simulink model "controller_dev_sg"  (R2018b)
settings: configuration reference "Physics" (kept outside this file)
model workspace (MAT data in the model file):
  m = 1000
undefined symbols (not defined in the file or in its folder): C, P_MLOC_NumberOfNoSendFrames, tS, TUMHealthStatus, TUMStateEstimationState, TUMVehicleState, x0_vehiclepose_stm
libraries: xpcrtudplib x13, simulink x12, canmsglib x12, etargetslib x10, speedgoatlib_IO614 x9, misc x4, xpcutilitieslib x1
(part 1 of 2)
settings Model: DataDictionary=controller_dev_sg.sldd  sg_rtwmakecfg_data=_sglibc__IO61X_Library_  PauseTimes=9.280  Creator=wischnewski  LastModifiedBy=ge34qer

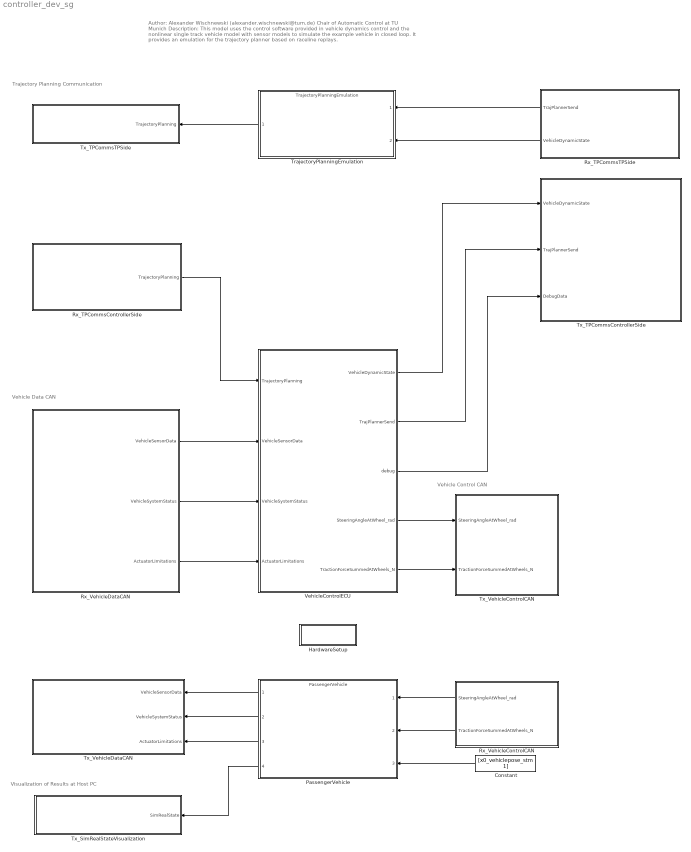
== system controller_dev_sg ==
  note: Visualization of Results at Host PC
  note: Trajectory Planning Communication
  note: Vehicle Control CAN
  note: Vehicle Data CAN
  note: Author: Alexander Wischnewski (alexander.wischnewski@tum.de)
      | Chair of Automatic Control at TU Munich
      |
      | Description: This model uses the control software provided in vehicle dynamics control and the nonlinear single track vehicle model
      | with sensor models to simulate the example vehicle in closed loop. It provides an emulation for the trajectory planner based on raceline replays.
  Constant : Constant  Value=[x0_vehiclepose_stm 1]
  HardwareSetup : Subsystem
  PassengerVehicle : ModelReference  ModelNameDialog=PassengerVehicle  SimulationMode=Normal  ModelReferenceVersion=1.770
  Rx_TPCommsControllerSide : Subsystem
  Rx_TPCommsTPSide : Subsystem
  Rx_VehicleControlCAN : Subsystem
  Rx_VehicleDataCAN : Subsystem
  TrajectoryPlanningEmulation : ModelReference  ModelNameDialog=TrajectoryPlanningEmulation.slx  SimulationMode=Normal  ModelReferenceVersion=1.722
  Tx_SimRealStateVisualization : Subsystem
  Tx_TPCommsControllerSide : Subsystem
  Tx_TPCommsTPSide : Subsystem
  Tx_VehicleControlCAN : Subsystem
  Tx_VehicleDataCAN : Subsystem
  VehicleControlECU : Subsystem
  wires:
  VehicleControlECU/3(debug) -> Tx_TPCommsControllerSide/3(DebugData)
  Rx_TPCommsControllerSide/1(TrajectoryPlanning) -> VehicleControlECU/1(TrajectoryPlanning)
  VehicleControlECU/1(VehicleDynamicState) -> Tx_TPCommsControllerSide/1(VehicleDynamicState)
  VehicleControlECU/2(TrajPlannerSend) -> Tx_TPCommsControllerSide/2(TrajPlannerSend)
  Rx_TPCommsTPSide/1(TrajPlannerSend) -> TrajectoryPlanningEmulation/1
  Rx_TPCommsTPSide/2(VehicleDynamicState) -> TrajectoryPlanningEmulation/2
  TrajectoryPlanningEmulation/1 -> Tx_TPCommsTPSide/1(TrajectoryPlanning)
  VehicleControlECU/4(SteeringAngleAtWheel_rad) -> Tx_VehicleControlCAN/1(SteeringAngleAtWheel_rad)
  VehicleControlECU/5(TractionForceSummedAtWheels_N) -> Tx_VehicleControlCAN/2(TractionForceSummedAtWheels_N)
  Rx_VehicleControlCAN/1(SteeringAngleAtWheel_rad) -> PassengerVehicle/1
  Rx_VehicleControlCAN/2(TractionForceSummedAtWheels_N) -> PassengerVehicle/2
  PassengerVehicle/1 -> Tx_VehicleDataCAN/1(VehicleSensorData)
  PassengerVehicle/2 -> Tx_VehicleDataCAN/2(VehicleSystemStatus)
  PassengerVehicle/3 -> Tx_VehicleDataCAN/3(ActuatorLimitations)
  Rx_VehicleDataCAN/3(ActuatorLImitations) -> VehicleControlECU/4(ActuatorLimitations)
  Rx_VehicleDataCAN/2(VehicleSystemStatus) -> VehicleControlECU/3(VehicleSystemStatus)
  Rx_VehicleDataCAN/1(VehicleSensorData) -> VehicleControlECU/2(VehicleSensorData)
  PassengerVehicle/4 -> Tx_SimRealStateVisualization/1(SimRealState)
  Constant/1 -> PassengerVehicle/3

== system controller_dev_sg/HardwareSetup ==
  CAN & LIN Setup : speedgoatlib_IO614/CAN & LIN Setup  id=1  drLtr=C:  PCISlot=-1  port1=CAN (HS/LS)  port2=CAN (HS)  port3=CAN (HS)  port4=CAN (HS)  opModeCAN1=Highspeed (HS)  bdrCAN1=1 MBaud  usrBdrCAN1=[5, 1, 13, 2]  stdAccMaskCAN1=[0, 0]  extAccMaskCAN1=[0, 0]  opModeCAN2=Highspeed (HS)  bdrCAN2=1 MBaud  usrBdrCAN2=[5, 1, 13, 2]  stdAccMaskCAN2=[0, 0]  extAccMaskCAN2=[0, 0]  opModeCAN3=Highspeed (HS)  bdrCAN3=1 MBaud  usrBdrCAN3=[5, 1, 13, 2]  stdAccMaskCAN3=[0, 0]  extAccMaskCAN3=[0, 0]  opModeCAN4=Highspeed (HS)  bdrCAN4=1 MBaud  usrBdrCAN4=[5, 1, 13, 2]  stdAccMaskCAN4=[0, 0]  extAccMaskCAN4=[0, 0]  initStruct=[]  termStruct=[]  opModeLIN=Master  bdrLIN=19200  protl=IO614  qtyMod=1  chNo=[1, 2, 3, 4]  ptTypes=[1, 1, 1, 1, 2]  protlHelpIdx=[0, 1, 2, 3, 0]  isFDMod=0  drvLtr=C:  opModeLIN2=Master  bdrLIN2=19200
      settings: SourceProductName=Simulink Real-Time: Speedgoat Library
  "Real-time UDP Configuration " : xpcrtudplib/UDP Configure  Priority=1  IpAddress=10.0.1.0  SubnetMask=255.255.255.0  Gateway=0.0.0.0  PciBus=14  PciSlot=0  PciFunction=0  ID=3  tune=0  disable=off  enableMulticast=off  MulticastIpAddress={}  MulticastMask={}
      settings: SourceProductName=Simulink Real-Time  SourceProductBaseCode=XP
  Real-time UDP Configuration 1 : xpcrtudplib/UDP Configure  Priority=1  IpAddress=10.0.2.0  SubnetMask=255.255.255.0  Gateway=0.0.0.0  PciBus=16  PciSlot=0  PciFunction=0  ID=3  tune=0  disable=off  enableMulticast=off  MulticastIpAddress={}  MulticastMask={}
      settings: SourceProductName=Simulink Real-Time  SourceProductBaseCode=XP

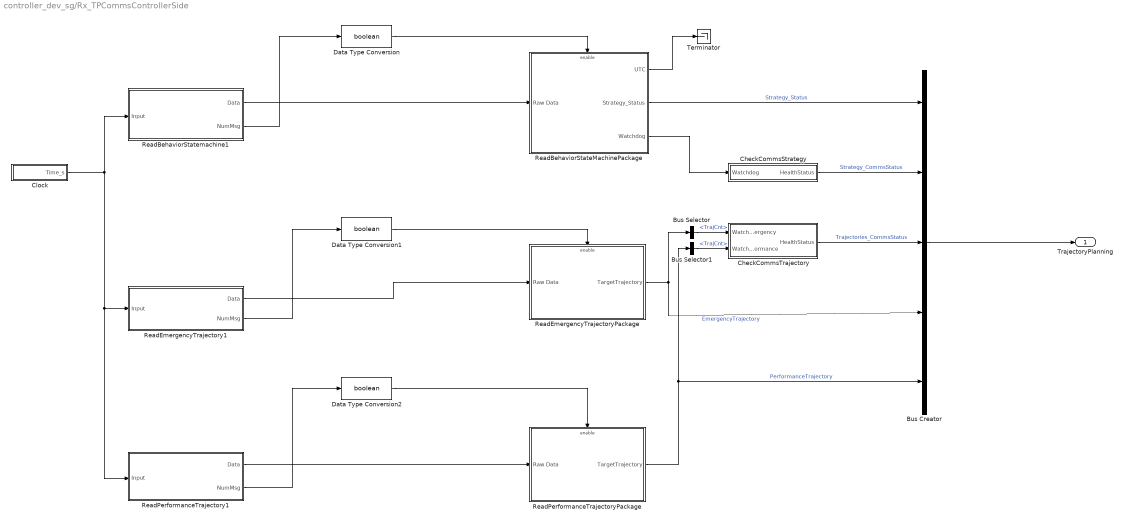
== system controller_dev_sg/Rx_TPCommsControllerSide ==
  Bus Creator : BusCreator  Inputs=5
  Bus Selector : BusSelector  OutputSignals=TrajCnt
  Bus Selector1 : BusSelector  OutputSignals=TrajCnt
  CheckCommsStrategy : Subsystem
  CheckCommsTrajectory : Subsystem
  Clock : Subsystem
  Data Type Conversion : DataTypeConversion  OutDataTypeStr=boolean
  Data Type Conversion1 : DataTypeConversion  OutDataTypeStr=boolean
  Data Type Conversion2 : DataTypeConversion  OutDataTypeStr=boolean
  ReadBehaviorStateMachinePackage : Subsystem  Priority=1000
  ReadBehaviorStatemachine1 : Subsystem  Priority=1
  ReadEmergencyTrajectory1 : Subsystem  Priority=1000
  ReadEmergencyTrajectoryPackage : Subsystem  Priority=1000
  ReadPerformanceTrajectory1 : Subsystem  Priority=1000
  ReadPerformanceTrajectoryPackage : Subsystem  Priority=1000
  Terminator : Terminator
  TrajectoryPlanning : Outport  OutDataTypeStr=Bus: TrajectoryPlanning  BusOutputAsStruct=on
  wires:
  ReadBehaviorStateMachinePackage/1(UTC) -> Terminator/1
  ReadPerformanceTrajectoryPackage/1(TargetTrajectory) -> Bus Selector1/1, Bus Creator/5  "PerformanceTrajectory"
  Clock/1(Time_s) -> ReadPerformanceTrajectory1/1(Input), ReadEmergencyTrajectory1/1(Input), ReadBehaviorStatemachine1/1(Input)
  CheckCommsTrajectory/1(HealthStatus) -> Bus Creator/3  "Trajectories_CommsStatus"
  ReadBehaviorStateMachinePackage/2(Strategy_Status) -> Bus Creator/1  "Strategy_Status"
  CheckCommsStrategy/1(HealthStatus) -> Bus Creator/2  "Strategy_CommsStatus"
  ReadEmergencyTrajectoryPackage/1(TargetTrajectory) -> Bus Creator/4, Bus Selector/1  "EmergencyTrajectory"
  Bus Selector/1 -> CheckCommsTrajectory/1(WatchdogEmergency)  "<TrajCnt>"
  Bus Selector1/1 -> CheckCommsTrajectory/2(WatchdogPerformance)  "<TrajCnt>"
  ReadBehaviorStateMachinePackage/3(Watchdog) -> CheckCommsStrategy/1(Watchdog)
  ReadEmergencyTrajectory1/2(NumMsg) -> Data Type Conversion1/1
  ReadEmergencyTrajectory1/1(Data) -> ReadEmergencyTrajectoryPackage/1(Raw Data)
  ReadPerformanceTrajectory1/1(Data) -> ReadPerformanceTrajectoryPackage/1(Raw Data)
  ReadPerformanceTrajectory1/2(NumMsg) -> Data Type Conversion2/1
  ReadBehaviorStatemachine1/2(NumMsg) -> Data Type Conversion/1
  ReadBehaviorStatemachine1/1(Data) -> ReadBehaviorStateMachinePackage/1(Raw Data)
  Data Type Conversion/1 -> ReadBehaviorStateMachinePackage/Enable
  Data Type Conversion1/1 -> ReadEmergencyTrajectoryPackage/Enable
  Data Type Conversion2/1 -> ReadPerformanceTrajectoryPackage/Enable
  Bus Creator/1 -> TrajectoryPlanning/1

== system controller_dev_sg/Rx_TPCommsTPSide ==
  Bus Creator : BusCreator  Inputs=2
  Data Type Conversion : DataTypeConversion  OutDataTypeStr=boolean
  Data Type Conversion1 : DataTypeConversion  OutDataTypeStr=boolean
  ReadBehaviorStateMachine : Subsystem  Priority=1000
  ReadBehaviorStateMachinePackage : Subsystem  Priority=1000
  ReadTrajectoryGeneration : Subsystem  Priority=1000
  ReadTrajectoryGeneration1 : Subsystem  Priority=1000
  Subsystem : Subsystem
  Terminator : Terminator
  TrajPlannerSend : Outport  OutDataTypeStr=Bus: TrajPlanner_Send
  VehicleDynamicState : Outport  Port=2  OutDataTypeStr=Bus: VehicleDynamicState
  wires:
  ReadBehaviorStateMachinePackage/1(TUMVehicleState) -> Bus Creator/1  "TUMVehicleState"
  Bus Creator/1 -> TrajPlannerSend/1
  ReadTrajectoryGeneration1/1(BDriveMode) -> Bus Creator/2  "BDriveMode"
  ReadBehaviorStateMachinePackage/2(ErrorCode) -> Terminator/1
  Data Type Conversion/1 -> ReadBehaviorStateMachinePackage/Enable
  Data Type Conversion1/1 -> ReadTrajectoryGeneration1/Enable
  ReadBehaviorStateMachine/2(NumMsg) -> Data Type Conversion/1
  ReadBehaviorStateMachine/1(Data) -> ReadBehaviorStateMachinePackage/1(Raw Data)
  ReadTrajectoryGeneration/1(Data) -> ReadTrajectoryGeneration1/1(Raw Data)
  ReadTrajectoryGeneration/2(NumMsg) -> Data Type Conversion1/1
  ReadTrajectoryGeneration1/2(RcvData) -> Subsystem/1(RcvData)
  Subsystem/1(VehicleDynamicState) -> VehicleDynamicState/1

== system controller_dev_sg/Rx_VehicleControlCAN ==
  CAN Read : speedgoatlib_IO614/CAN/CAN Read  id=1  sampleTime=-1  portSelection=2  messageType=CAN  protl=IO614  ptIdx=1  isFDMod=0
      settings: SourceProductName=Simulink Real-Time: Speedgoat Library
  CAN Unpack : canmsglib/CAN Unpack  MsgList=(none)  MsgName=CAN Msg  MsgIDType=Standard (11-bit identifier)  MsgIdentifier=24  MsgLength=8  SignalInfo=SteeringAngleAtWheel_rad$0$24$1$1$1$0$0.000001$0$-Inf$Inf$#TractionforceSummedAtWheels_N$24$24$1$1$1$0$0.01$0$-Inf$Inf$#  NSignals=2  IDPort=off  TimestampPort=off  ErrorPort=off  RemotePort=off  LengthPort=off  StatusPort=off  StartBits=str2num('[int32(0);int32(24)]')  SignalSizes=str2num('[int32(24);int32(24)]')  ByteOrders=str2num('[int32(1);int32(1)]')  DataTypes=str2num('[int32(1);int32(1)]')  MultiplexTypes=str2num('[int32(1);int32(1)]')  MultiplexValues=str2num('[double(0);double(0)]')  Factors=str2num('[double(0.000001);double(0.01)]')  Offsets=str2num('[double(0);double(0)]')  Minimums=str2num('[double(-Inf);double(-Inf)]')  Maximums=str2num('[double(Inf);double(Inf)]')  ApplyMinMax=off
      settings: SourceProductName=Simulink Real-Time
  While Iterator : WhileIterator  MaxIters=501  WhileBlockType=do-while
  SteeringAngleAtWheel_rad : Outport
  TractionForceSummedAtWheels_N : Outport  Port=2
  wires:
  CAN Unpack/2 -> TractionForceSummedAtWheels_N/1
  CAN Unpack/1 -> SteeringAngleAtWheel_rad/1
  CAN Read/2 -> CAN Unpack/1
  CAN Read/1 -> While Iterator/1

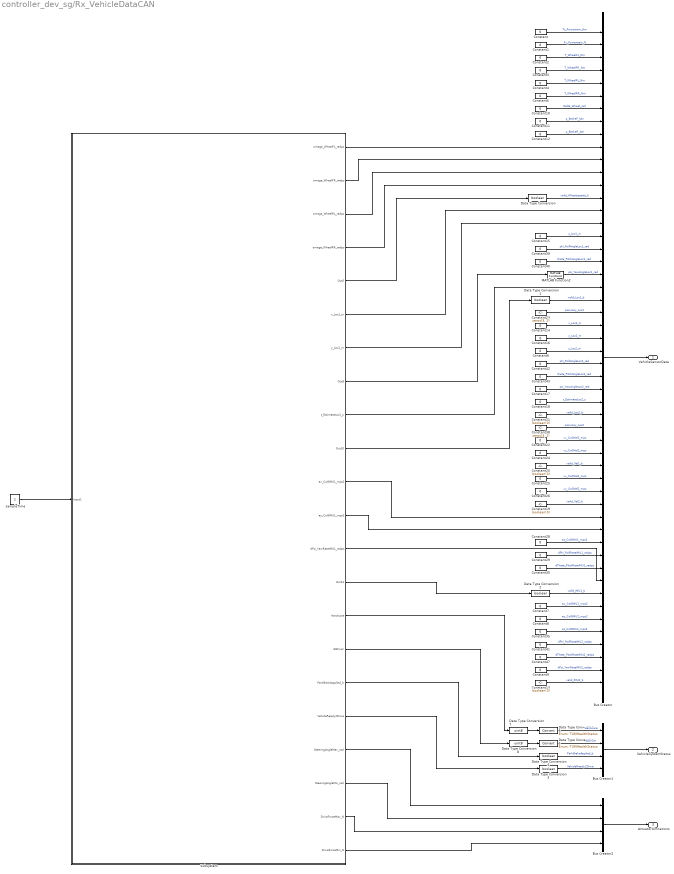
== system controller_dev_sg/Rx_VehicleDataCAN ==
  Bus Creator : BusCreator  Inputs=52  OutDataTypeStr=Bus: VehicleSensorData
  Bus Creator1 : BusCreator  Inputs=4  OutDataTypeStr=Bus: VehicleSystemStatus
  Bus Creator2 : BusCreator  Inputs=4  OutDataTypeStr=Bus: ActuatorLimitations
  Constant{,1..12,14..18,22,24..26,28..30,35,39..43,47} (32 alike) : Constant  Value=0
  Constant{13,19..21} (4 alike) : Constant  Value=boolean(0)
  Constant23 : Constant  Value=zeros(3, 1)
  Constant38 : Constant  Value=zeros(3, 1)
  Data Type Conversion{,1..4} (5 alike) : DataTypeConversion  OutDataTypeStr=boolean
  Data Type Conversion5 : DataTypeConversion  OutDataTypeStr=Enum: TUMHealthStatus
  Data Type Conversion6 : DataTypeConversion  OutDataTypeStr=Enum: TUMHealthStatus
  Data Type Conversion7 : DataTypeConversion  OutDataTypeStr=uint8
  Data Type Conversion8 : DataTypeConversion  OutDataTypeStr=uint8
  MATLAB Function2 : misc/MATLAB Function2  SystemSampleTime=-1
  Subsystem : Subsystem
  sampleTime : Constant  SampleTime=tS
  VehicleSensorData : Outport  OutDataTypeStr=Bus: VehicleSensorData
  VehicleSystemStatus : Outport  Port=2  OutDataTypeStr=Bus: VehicleSystemStatus
  ActuatorLImitations : Outport  Port=3  OutDataTypeStr=Bus: ActuatorLimitations
  wires:
  Constant30/1 -> Bus Creator/43  "dTheta_PitchRateIMU1_radps"
  Constant12/1 -> Bus Creator/9  "p_BrakeR_bar"
  Constant5/1 -> Bus Creator/6  "T_WheelRR_Nm"
  Constant1/1 -> Bus Creator/2  "Fx_Powertrain_N"
  Constant19/1 -> Bus Creator/38  "valid_Vel2_b"
  Constant7/1 -> Bus Creator/46  "ax_CoGIMU2_mps2"
  Constant11/1 -> Bus Creator/8  "p_BrakeF_bar"
  Bus Creator/1 -> VehicleSensorData/1
  Constant21/1 -> Bus Creator/31  "valid_Loc2_b"
  Constant/1 -> Bus Creator/1  "Tz_Powertrain_Nm"
  Constant25/1 -> Bus Creator/36  "vx_CoGVel2_mps"
  Constant38/1 -> Bus Creator/32  "accuracy_Loc2"
  Constant8/1 -> Bus Creator/47  "ay_CoGIMU2_mps2"
  Constant3/1 -> Bus Creator/4  "T_WheelFR_Nm"
  Constant10/1 -> Bus Creator/7  "Delta_Wheel_rad"
  Constant14/1 -> Bus Creator/24  "x_Loc2_m"
  Constant40/1 -> Bus Creator/19  "theta_PitchAngleLoc1_rad"
  Constant23/1 -> Bus Creator/23  "accuracy_Loc1"
  Constant4/1 -> Bus Creator/5  "T_WheelRL_Nm"
  Constant28/1 -> Bus Creator/41  "az_CoGIMU1_mps2"
  Constant20/1 -> Bus Creator/35  "valid_Vel1_b"
  Constant6/1 -> Bus Creator/26  "z_Loc2_m"
  Constant2/1 -> Bus Creator/3  "T_WheelFL_Nm"
  Constant39/1 -> Bus Creator/18  "phi_RollAngleLoc1_rad"
  Constant15/1 -> Bus Creator/17  "z_Loc1_m"
  Constant26/1 -> Bus Creator/37  "vy_CoGVel2_mps"
  Constant16/1 -> Bus Creator/25  "y_Loc2_m"
  MATLAB Function2/1 -> Bus Creator/20  "psi_YawAngleLoc1_rad"
  Constant42/1 -> Bus Creator/27  "phi_RollAngleLoc2_rad"
  Constant9/1 -> Bus Creator/51  "dPsi_YawRateIMU2_radps"
  Constant17/1 -> Bus Creator/29  "psi_YawAngleLoc2_rad"
  Constant24/1 -> Bus Creator/34  "vy_CoGVel1_mps"
  Constant13/1 -> Bus Creator/52  "valid_IMU2_b"
  Constant29/1 -> Bus Creator/42  "dPhi_RollRateIMU1_radps"
  Constant22/1 -> Bus Creator/33  "vx_CoGVel1_mps"
  Constant18/1 -> Bus Creator/30  "t_EstimateLoc2_s"
  Constant43/1 -> Bus Creator/28  "theta_PitchAngleLoc2_rad"
  Constant47/1 -> Bus Creator/50  "dTheta_PitchRateIMU2_radps"
  Constant41/1 -> Bus Creator/49  "dPhi_RollRateIMU2_radps"
  Constant35/1 -> Bus Creator/48  "az_CoGIMU2_mps2"
  Bus Creator1/1 -> VehicleSystemStatus/1
  Bus Creator2/1 -> ActuatorLImitations/1
  Data Type Conversion/1 -> Bus Creator/14  "valid_Wheelspeeds_b"
  Data Type Conversion1/1 -> Bus Creator/22  "valid_Loc1_b"
  Data Type Conversion2/1 -> Bus Creator/45  "valid_IMU1_b"
  Data Type Conversion3/1 -> Bus Creator1/4  "VehicleReady2Drive"
  Data Type Conversion4/1 -> Bus Creator1/3  "ParkBrakeApplied_b"
  Data Type Conversion5/1 -> Bus Creator1/2  "AIDriver"
  Data Type Conversion6/1 -> Bus Creator1/1  "Hardware"
  Data Type Conversion7/1 -> Data Type Conversion6/1
  Data Type Conversion8/1 -> Data Type Conversion5/1
  Subsystem/1(omega_WheelFL_radps) -> Bus Creator/10
  Subsystem/2(omega_WheelFR_radps) -> Bus Creator/11
  Subsystem/3(omega_WheelRL_radps) -> Bus Creator/12
  Subsystem/4(omega_WheelRR_radps) -> Bus Creator/13
  Subsystem/5(Out5) -> Data Type Conversion/1
  Subsystem/6(x_Loc1_m) -> Bus Creator/15
  Subsystem/7(y_Loc1_m) -> Bus Creator/16
  Subsystem/8(Out8) -> MATLAB Function2/1
  Subsystem/9(t_EstimateLoc1_s) -> Bus Creator/21
  Subsystem/10(Out10) -> Data Type Conversion1/1
  Subsystem/11(ax_CoGIMU1_mps2) -> Bus Creator/39
  Subsystem/12(ay_CoGIMU1_mps2) -> Bus Creator/40
  Subsystem/13(dPsi_YawRateIMU1_radps) -> Bus Creator/44
  Subsystem/14(Out14) -> Data Type Conversion2/1
  Subsystem/15(Hardware) -> Data Type Conversion7/1
  Subsystem/16(AIDriver) -> Data Type Conversion8/1
  Subsystem/17(ParkBrakeApplied_b) -> Data Type Conversion4/1
  Subsystem/18(VehicleReady2Drive) -> Data Type Conversion3/1
  Subsystem/19(SteeringAngleMax_rad) -> Bus Creator2/1
  Subsystem/20(SteeringAngleMin_rad) -> Bus Creator2/2
  Subsystem/21(DriveForceMax_N) -> Bus Creator2/3
  Subsystem/22(DriveForceMin_N) -> Bus Creator2/4
  sampleTime/1 -> Subsystem/1(Input1)

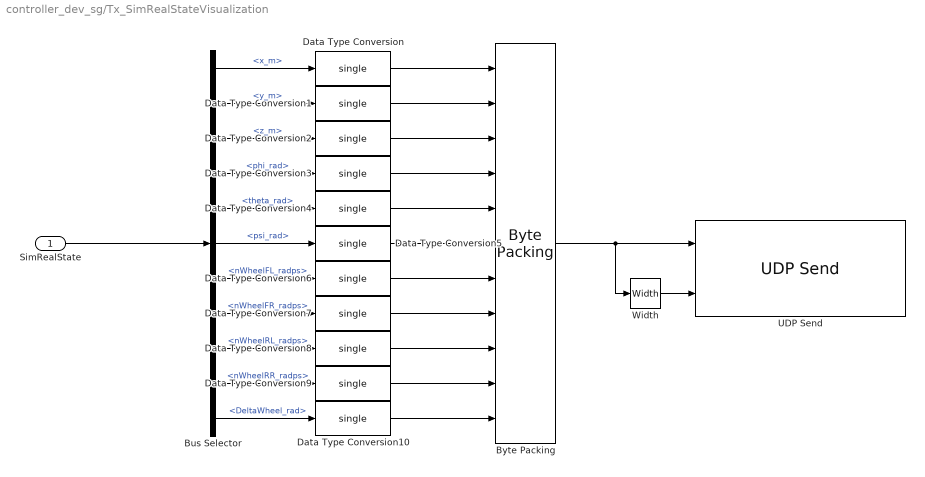
== system controller_dev_sg/Tx_SimRealStateVisualization ==
  SimRealState : Inport
  Bus Selector : BusSelector  OutputSignals=x_m,y_m,z_m,phi_rad,theta_rad,psi_rad,nWheelFL_radps,nWheelFR_radps,nWheelRL_radps,nWheelRR_radps,DeltaWheel_rad
  "Byte Packing " : xpcutilitieslib/Byte Packing   MaskPackedDataType=uint8  MaskUnpackedDataTypes={'single','single','single','single','single','single','single','single','single','single','single'}  MaskAlignment=1
  Data Type Conversion{,1..10} (11 alike) : DataTypeConversion  OutDataTypeStr=single
  UDP Send : xpcrtudplib/UDP Send  ipAddressVal=Use host-target connection  localPort=-1  toAddress=192.168.7.2  toPort=25000  sampleTime=-1
      settings: SourceProductName=Simulink Real-Time  SourceProductBaseCode=XP
  Width : Width
  wires:
  SimRealState/1 -> Bus Selector/1
  Bus Selector/1 -> Data Type Conversion/1  "<x_m>"
  Bus Selector/2 -> Data Type Conversion1/1  "<y_m>"
  Bus Selector/3 -> Data Type Conversion2/1  "<z_m>"
  Bus Selector/4 -> Data Type Conversion3/1  "<phi_rad>"
  Bus Selector/5 -> Data Type Conversion4/1  "<theta_rad>"
  Bus Selector/6 -> Data Type Conversion5/1  "<psi_rad>"
  Bus Selector/7 -> Data Type Conversion6/1  "<nWheelFL_radps>"
  Bus Selector/8 -> Data Type Conversion7/1  "<nWheelFR_radps>"
  Bus Selector/9 -> Data Type Conversion8/1  "<nWheelRL_radps>"
  Bus Selector/10 -> Data Type Conversion9/1  "<nWheelRR_radps>"
  Bus Selector/11 -> Data Type Conversion10/1  "<DeltaWheel_rad>"
  Data Type Conversion/1 -> "Byte Packing "/1
  Data Type Conversion1/1 -> "Byte Packing "/2
  Data Type Conversion2/1 -> "Byte Packing "/3
  Data Type Conversion3/1 -> "Byte Packing "/4
  Data Type Conversion4/1 -> "Byte Packing "/5
  Data Type Conversion5/1 -> "Byte Packing "/6
  Data Type Conversion6/1 -> "Byte Packing "/7
  Data Type Conversion7/1 -> "Byte Packing "/8
  Data Type Conversion8/1 -> "Byte Packing "/9
  Data Type Conversion9/1 -> "Byte Packing "/10
  Data Type Conversion10/1 -> "Byte Packing "/11
  "Byte Packing "/1 -> Width/1, UDP Send/1
  Width/1 -> UDP Send/2

== system controller_dev_sg/Tx_TPCommsControllerSide ==
  VehicleDynamicState : Inport
  TrajPlannerSend : Inport  Port=2
  DebugData : Inport  Port=3
  BehaviorStatemachine : Subsystem
  Digital Clock : DigitalClock  SampleTime=-1
  SendToBehaviorStatemachine1 : Subsystem
  SendToTrajectoryGeneration1 : Subsystem
  TrajectoryGeneration : Subsystem
  wires:
  DebugData/1 -> BehaviorStatemachine/2(DebugData)
  TrajPlannerSend/1 -> TrajectoryGeneration/1(TrajPlannerSend), BehaviorStatemachine/1(TrajPlannerSend)
  VehicleDynamicState/1 -> TrajectoryGeneration/2(VehicleDynamicState)
  Digital Clock/1 -> TrajectoryGeneration/3(Time_s)
  BehaviorStatemachine/2(BSM_Package) -> SendToBehaviorStatemachine1/1(Data)  "BSM_Package"
  TrajectoryGeneration/2(TG_Package) -> SendToTrajectoryGeneration1/1(Data)
  TrajectoryGeneration/1(TG_ActivateSend) -> SendToTrajectoryGeneration1/Enable  "TG_ActivateSend"
  BehaviorStatemachine/1(BSM_ActivateSend) -> SendToBehaviorStatemachine1/Enable  "BSM_ActivateSend"

== system controller_dev_sg/Tx_TPCommsTPSide ==
  TrajectoryPlanning : Inport
  BSM_Package : Subsystem
  EmergencyTrajectory : Subsystem
  PerformanceTrajectory : Subsystem
  SendBehaviorStateMachine : Subsystem
  SendEmergencyTrajectory : Subsystem
  SendPerformanceTrajectory : Subsystem
  wires:
  TrajectoryPlanning/1 -> BSM_Package/1(TrajPlannerSend), PerformanceTrajectory/1(TrajPlannerSend), EmergencyTrajectory/1(TrajPlannerSend)
  EmergencyTrajectory/2(EMT_Package) -> SendEmergencyTrajectory/1(Data)
  PerformanceTrajectory/2(PMT_Package) -> SendPerformanceTrajectory/1(Data)
  BSM_Package/2(BSM_Package) -> SendBehaviorStateMachine/1(Data)
  BSM_Package/1(BSM_ActivateSend) -> SendBehaviorStateMachine/Enable
  PerformanceTrajectory/1(PMT_ActivateSend) -> SendPerformanceTrajectory/Enable
  EmergencyTrajectory/1(EMT_ActivateSend) -> SendEmergencyTrajectory/Enable

== system controller_dev_sg/Tx_VehicleControlCAN ==
  SteeringAngleAtWheel_rad : Inport
  TractionForceSummedAtWheels_N : Inport  Port=2
  "CAN Pack " : canmsglib/CAN Pack  MsgList=(none)  MsgName=CAN Msg  MsgIDType=Standard (11-bit identifier)  MsgIdentifier=24  MsgLength=8  SignalInfo=SteeringAngleAtWheel_rad$0$24$1$1$1$0$0.000001$0$-Inf$Inf$#TractionForceSummedAtWheels_N$24$24$1$1$1$0$0.01$0$-Inf$Inf$#  NSignals=2  StartBits=str2num('[int32(0);int32(24)]')  SignalSizes=str2num('[int32(24);int32(24)]')  ByteOrders=str2num('[int32(1);int32(1)]')  DataTypes=str2num('[int32(1);int32(1)]')  MultiplexTypes=str2num('[int32(1);int32(1)]')  MultiplexValues=str2num('[double(0);double(0)]')  Factors=str2num('[double(0.000001);double(0.01)]')  Offsets=str2num('[double(0);double(0)]')  Minimums=str2num('[double(-Inf);double(-Inf)]')  Maximums=str2num('[double(Inf);double(Inf)]')  Remote=off  ApplyMinMax=off  BusOutput=off
      settings: SourceProductName=Simulink Real-Time  DataFormat=manually specified signals
  CAN Write : speedgoatlib_IO614/CAN/CAN Write  id=1  sampleTime=-1  portSelection=1  messageType=CAN  enaStatusPort=off  protl=IO614  ptIdx=0  isFDMod=0
      settings: SourceProductName=Simulink Real-Time: Speedgoat Library
  wires:
  "CAN Pack "/1 -> CAN Write/1
  TractionForceSummedAtWheels_N/1 -> "CAN Pack "/2
  SteeringAngleAtWheel_rad/1 -> "CAN Pack "/1

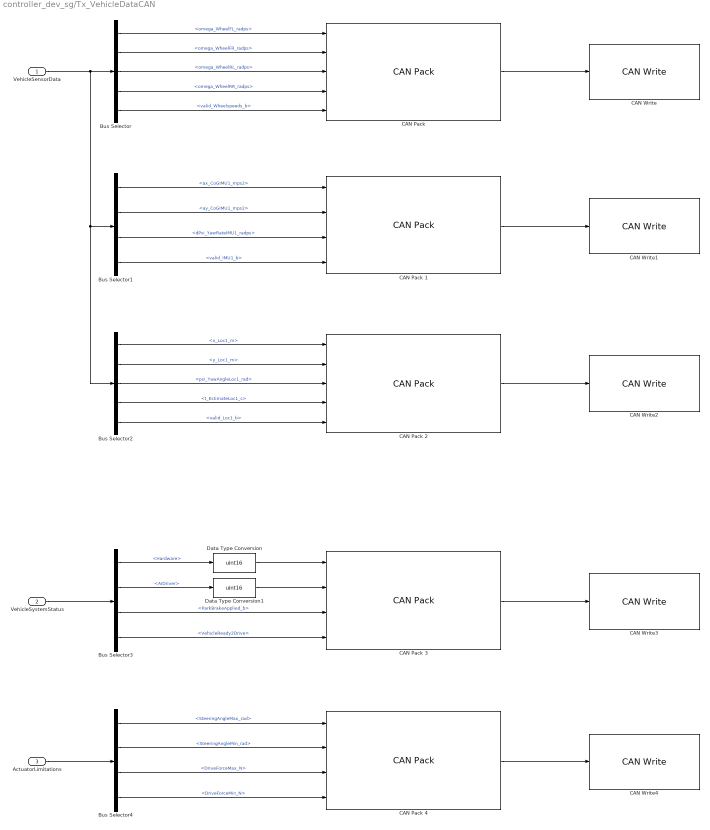
== system controller_dev_sg/Tx_VehicleDataCAN ==
  VehicleSensorData : Inport
  VehicleSystemStatus : Inport  Port=2
  ActuatorLimitations : Inport  Port=3
  Bus Selector : BusSelector  OutputSignals=omega_WheelFL_radps,omega_WheelFR_radps,omega_WheelRL_radps,omega_WheelRR_radps,valid_Wheelspeeds_b
  Bus Selector1 : BusSelector  OutputSignals=ax_CoGIMU1_mps2,ay_CoGIMU1_mps2,dPsi_YawRateIMU1_radps,valid_IMU1_b
  Bus Selector2 : BusSelector  OutputSignals=x_Loc1_m,y_Loc1_m,psi_YawAngleLoc1_rad,t_EstimateLoc1_s,valid_Loc1_b
  Bus Selector3 : BusSelector  OutputSignals=Hardware,AIDriver,ParkBrakeApplied_b,VehicleReady2Drive
  Bus Selector4 : BusSelector  OutputSignals=SteeringAngleMax_rad,SteeringAngleMin_rad,DriveForceMax_N,DriveForceMin_N
  "CAN Pack " : canmsglib/CAN Pack  MsgList=(none)  MsgName=CAN Msg  MsgIDType=Standard (11-bit identifier)  MsgIdentifier=768  MsgLength=8  SignalInfo=omega_WheelFL_radps$0$15$1$1$1$0$0.1$0$-Inf$Inf$#omega_WheelFR_radps$15$15$1$1$1$0$0.1$0$-Inf$Inf$#omega_WheelRL_radps$30$15$1$1$1$0$0.1$0$-Inf$Inf$#omega_WheelRR_radps$45$15$1$1$1$0$0.1$0$-Inf$Inf$#valid_Wheelspeeds_b$60$4$1$1$1$0$1$0$-Inf$Inf$#  NSignals=5  StartBits=str2num('[int32(0);int32(15);int32(30);int32(45);int32(60)]')  SignalSizes=str2num('[int32(15);int32(15);int32(15);int32(15);int32(4)]')  ByteOrders=str2num('[int32(1);int32(1);int32(1);int32(1);int32(1)]')  DataTypes=str2num('[int32(1);int32(1);int32(1);int32(1);int32(1)]')  MultiplexTypes=str2num('[int32(1);int32(1);int32(1);int32(1);int32(1)]')  MultiplexValues=str2num('[double(0);double(0);double(0);double(0);double(0)]')  Factors=str2num('[double(0.1);double(0.1);double(0.1);double(0.1);double(1)]')  Offsets=str2num('[double(0);double(0);double(0);double(0);double(0)]')  Minimums=str2num('[double(-Inf);double(-Inf);double(-Inf);double(-Inf);double(-Inf)]')  Maximums=str2num('[double(Inf);double(Inf);double(Inf);double(Inf);double(Inf)]')  Remote=off  ApplyMinMax=off  BusOutput=off
      settings: SourceProductName=Simulink Real-Time  DataFormat=manually specified signals
  CAN Pack 1 : canmsglib/CAN Pack  MsgList=(none)  MsgName=CAN Msg  MsgIDType=Standard (11-bit identifier)  MsgIdentifier=48  MsgLength=8  SignalInfo=ax_CoGIMU1_mps2$0$16$1$1$1$0$0.001$0$-Inf$Inf$#ay_CoGIMU1_mps2$16$16$1$1$1$0$0.001$0$-Inf$Inf$#dPsi_YawRateIMU1_radps$32$16$1$1$1$0$0.0001$0$-Inf$Inf$#valid_IMU1_b$48$16$1$1$1$0$1$0$-Inf$Inf$#  NSignals=4  StartBits=str2num('[int32(0);int32(16);int32(32);int32(48)]')  SignalSizes=str2num('[int32(16);int32(16);int32(16);int32(16)]')  ByteOrders=str2num('[int32(1);int32(1);int32(1);int32(1)]')  DataTypes=str2num('[int32(1);int32(1);int32(1);int32(1)]')  MultiplexTypes=str2num('[int32(1);int32(1);int32(1);int32(1)]')  MultiplexValues=str2num('[double(0);double(0);double(0);double(0)]')  Factors=str2num('[double(0.001);double(0.001);double(0.0001);double(1)]')  Offsets=str2num('[double(0);double(0);double(0);double(0)]')  Minimums=str2num('[double(-Inf);double(-Inf);double(-Inf);double(-Inf)]')  Maximums=str2num('[double(Inf);double(Inf);double(Inf);double(Inf)]')  Remote=off  ApplyMinMax=off  BusOutput=off
      settings: SourceProductName=Simulink Real-Time  DataFormat=manually specified signals
  CAN Pack 2 : canmsglib/CAN Pack  MsgList=(none)  MsgName=CAN Msg  MsgIDType=Standard (11-bit identifier)  MsgIdentifier=192  MsgLength=8  SignalInfo=x_Loc1_m$0$15$1$1$1$0$0.05$0$-Inf$Inf$#y_Loc1_m$15$15$1$1$1$0$0.05$0$-Inf$Inf$#psi_YawAngleLoc1_rad$30$15$1$1$1$0$0.001$0$-Inf$Inf$#t_EstimateLoc1_s$45$15$1$1$1$0$0.001$0$-Inf$Inf$#valid_Loc1_b$60$4$1$1$1$0$1$0$-Inf$Inf$#  NSignals=5  StartBits=str2num('[int32(0);int32(15);int32(30);int32(45);int32(60)]')  SignalSizes=str2num('[int32(15);int32(15);int32(15);int32(15);int32(4)]')  ByteOrders=str2num('[int32(1);int32(1);int32(1);int32(1);int32(1)]')  DataTypes=str2num('[int32(1);int32(1);int32(1);int32(1);int32(1)]')  MultiplexTypes=str2num('[int32(1);int32(1);int32(1);int32(1);int32(1)]')  MultiplexValues=str2num('[double(0);double(0);double(0);double(0);double(0)]')  Factors=str2num('[double(0.05);double(0.05);double(0.001);double(0.001);double(1)]')  Offsets=str2num('[double(0);double(0);double(0);double(0);double(0)]')  Minimums=str2num('[double(-Inf);double(-Inf);double(-Inf);double(-Inf);double(-Inf)]')  Maximums=str2num('[double(Inf);double(Inf);double(Inf);double(Inf);double(Inf)]')  Remote=off  ApplyMinMax=off  BusOutput=off
      settings: SourceProductName=Simulink Real-Time  DataFormat=manually specified signals
  CAN Pack 3 : canmsglib/CAN Pack  MsgList=(none)  MsgName=CAN Msg  MsgIDType=Standard (11-bit identifier)  MsgIdentifier=12  MsgLength=8  SignalInfo=Hardware$0$12$1$1$1$0$1$0$-Inf$Inf$#AIDriver$12$12$1$1$1$0$1$0$-Inf$Inf$#ParkBrakeApplied_b$24$12$1$1$1$0$1$0$-Inf$Inf$#VehicleReady2Drive$36$12$1$1$1$0$1$0$-Inf$Inf$#  NSignals=4  StartBits=str2num('[int32(0);int32(12);int32(24);int32(36)]')  SignalSizes=str2num('[int32(12);int32(12);int32(12);int32(12)]')  ByteOrders=str2num('[int32(1);int32(1);int32(1);int32(1)]')  DataTypes=str2num('[int32(1);int32(1);int32(1);int32(1)]')  MultiplexTypes=str2num('[int32(1);int32(1);int32(1);int32(1)]')  MultiplexValues=str2num('[double(0);double(0);double(0);double(0)]')  Factors=str2num('[double(1);double(1);double(1);double(1)]')  Offsets=str2num('[double(0);double(0);double(0);double(0)]')  Minimums=str2num('[double(-Inf);double(-Inf);double(-Inf);double(-Inf)]')  Maximums=str2num('[double(Inf);double(Inf);double(Inf);double(Inf)]')  Remote=off  ApplyMinMax=off  BusOutput=off
      settings: SourceProductName=Simulink Real-Time  DataFormat=manually specified signals
  CAN Pack 4 : canmsglib/CAN Pack  MsgList=(none)  MsgName=CAN Msg  MsgIDType=Standard (11-bit identifier)  MsgIdentifier=170  MsgLength=8  SignalInfo=SteeringAngleMax_rad$0$16$1$1$1$0$0.001$0$-Inf$Inf$#SteeringAngleMin_rad$16$16$1$1$1$0$0.001$0$-Inf$Inf$#DriveForceMax_N$32$16$1$1$1$0$100$0$-Inf$Inf$#DriveForceMin_N$48$16$1$1$1$0$100$0$-Inf$Inf$#  NSignals=4  StartBits=str2num('[int32(0);int32(16);int32(32);int32(48)]')  SignalSizes=str2num('[int32(16);int32(16);int32(16);int32(16)]')  ByteOrders=str2num('[int32(1);int32(1);int32(1);int32(1)]')  DataTypes=str2num('[int32(1);int32(1);int32(1);int32(1)]')  MultiplexTypes=str2num('[int32(1);int32(1);int32(1);int32(1)]')  MultiplexValues=str2num('[double(0);double(0);double(0);double(0)]')  Factors=str2num('[double(0.001);double(0.001);double(100);double(100)]')  Offsets=str2num('[double(0);double(0);double(0);double(0)]')  Minimums=str2num('[double(-Inf);double(-Inf);double(-Inf);double(-Inf)]')  Maximums=str2num('[double(Inf);double(Inf);double(Inf);double(Inf)]')  Remote=off  ApplyMinMax=off  BusOutput=off
      settings: SourceProductName=Simulink Real-Time  DataFormat=manually specified signals
  CAN Write{,1..4} (5 alike) : speedgoatlib_IO614/CAN/CAN Write  id=1  sampleTime=-1  portSelection=3  messageType=CAN  enaStatusPort=off  protl=IO614  ptIdx=2  isFDMod=0
      settings: SourceProductName=Simulink Real-Time: Speedgoat Library
  Data Type Conversion : DataTypeConversion  OutDataTypeStr=uint16
  Data Type Conversion1 : DataTypeConversion  OutDataTypeStr=uint16
  wires:
  Bus Selector/1 -> "CAN Pack "/1  "<omega_WheelFL_radps>"
  Bus Selector/2 -> "CAN Pack "/2  "<omega_WheelFR_radps>"
  Bus Selector/3 -> "CAN Pack "/3  "<omega_WheelRL_radps>"
  Bus Selector/4 -> "CAN Pack "/4  "<omega_WheelRR_radps>"
  Bus Selector/5 -> "CAN Pack "/5  "<valid_Wheelspeeds_b>"
  "CAN Pack "/1 -> CAN Write/1
  Bus Selector1/1 -> CAN Pack 1/1  "<ax_CoGIMU1_mps2>"
  Bus Selector1/2 -> CAN Pack 1/2  "<ay_CoGIMU1_mps2>"
  Bus Selector1/3 -> CAN Pack 1/3  "<dPsi_YawRateIMU1_radps>"
  Bus Selector1/4 -> CAN Pack 1/4  "<valid_IMU1_b>"
  CAN Pack 1/1 -> CAN Write1/1
  CAN Pack 2/1 -> CAN Write2/1
  VehicleSensorData/1 -> Bus Selector2/1, Bus Selector1/1, Bus Selector/1
  Bus Selector2/1 -> CAN Pack 2/1  "<x_Loc1_m>"
  Bus Selector2/2 -> CAN Pack 2/2  "<y_Loc1_m>"
  Bus Selector2/3 -> CAN Pack 2/3  "<psi_YawAngleLoc1_rad>"
  Bus Selector2/5 -> CAN Pack 2/5  "<valid_Loc1_b>"
  VehicleSystemStatus/1 -> Bus Selector3/1
  Bus Selector3/1 -> Data Type Conversion/1  "<Hardware>"
  Bus Selector3/2 -> Data Type Conversion1/1  "<AIDriver>"
  Bus Selector3/3 -> CAN Pack 3/3  "<ParkBrakeApplied_b>"
  Bus Selector3/4 -> CAN Pack 3/4  "<VehicleReady2Drive>"
  CAN Pack 3/1 -> CAN Write3/1
  CAN Pack 4/1 -> CAN Write4/1
  ActuatorLimitations/1 -> Bus Selector4/1
  Bus Selector4/1 -> CAN Pack 4/1  "<SteeringAngleMax_rad>"
  Bus Selector4/2 -> CAN Pack 4/2  "<SteeringAngleMin_rad>"
  Bus Selector4/3 -> CAN Pack 4/3  "<DriveForceMax_N>"
  Bus Selector4/4 -> CAN Pack 4/4  "<DriveForceMin_N>"
  Data Type Conversion/1 -> CAN Pack 3/1
  Data Type Conversion1/1 -> CAN Pack 3/2
  Bus Selector2/4 -> CAN Pack 2/4  "<t_EstimateLoc1_s>"

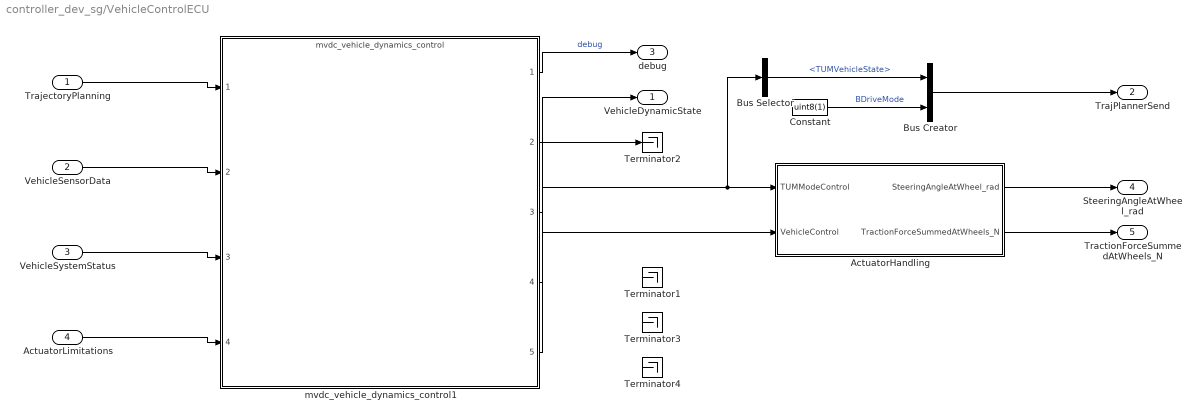
== system controller_dev_sg/VehicleControlECU ==
  TrajectoryPlanning : Inport
  VehicleSensorData : Inport  Port=2
  VehicleSystemStatus : Inport  Port=3
  ActuatorLimitations : Inport  Port=4
  ActuatorHandling : Subsystem
  Bus Creator : BusCreator  Inputs=2
  Bus Selector : BusSelector  OutputSignals=TUMVehicleState
  Constant : Constant  Value=uint8(1)
  Terminator{1..4} (4 alike) : Terminator
  mvdc_vehicle_dynamics_control1 : ModelReference  ModelNameDialog=mvdc_vehicle_dynamics_control  SimulationMode=Normal  ModelReferenceVersion=1.767
  VehicleDynamicState : Outport
  TrajPlannerSend : Outport  Port=2
  debug : Outport  Port=3
  SteeringAngleAtWheel_rad : Outport  Port=4
  TractionForceSummedAtWheels_N : Outport  Port=5
  wires:
  mvdc_vehicle_dynamics_control1/1 -> debug/1  "debug"
  VehicleSystemStatus/1 -> mvdc_vehicle_dynamics_control1/3
  ActuatorLimitations/1 -> mvdc_vehicle_dynamics_control1/4
  VehicleSensorData/1 -> mvdc_vehicle_dynamics_control1/2
  mvdc_vehicle_dynamics_control1/5 -> ActuatorHandling/2(VehicleControl)
  mvdc_vehicle_dynamics_control1/4 -> Bus Selector/1, ActuatorHandling/1(TUMModeControl)
  ? -> Terminator1/1
  mvdc_vehicle_dynamics_control1/3 -> Terminator2/1
  mvdc_vehicle_dynamics_control1/2 -> VehicleDynamicState/1
  ActuatorHandling/2(TractionForceSummedAtWheels_N) -> TractionForceSummedAtWheels_N/1
  ActuatorHandling/1(SteeringAngleAtWheel_rad) -> SteeringAngleAtWheel_rad/1
  ? -> Terminator3/1
  ? -> Terminator4/1
  Bus Selector/1 -> Bus Creator/1  "<TUMVehicleState>"
  Constant/1 -> Bus Creator/2  "BDriveMode"
  Bus Creator/1 -> TrajPlannerSend/1
  TrajectoryPlanning/1 -> mvdc_vehicle_dynamics_control1/1

== system controller_dev_sg/Rx_TPCommsControllerSide/CheckCommsStrategy ==
  Watchdog : Inport
  CheckComms : misc/CheckComms  timeout_s=tPX2CommsTimeout  tS=tS
  Constant1 : Constant  Value=TUMHealthStatus.ERROR  OutDataTypeStr=Enum: TUMHealthStatus
  Constant2 : Constant  Value=TUMHealthStatus.OK  OutDataTypeStr=Enum: TUMHealthStatus
  Switch1 : Switch  Criteria=u2 > Threshold
  HealthStatus : Outport
  wires:
  CheckComms/1 -> Switch1/2
  Constant2/1 -> Switch1/1
  Switch1/1 -> HealthStatus/1  "Strategy_CommsStatus"
  Constant1/1 -> Switch1/3
  Watchdog/1 -> CheckComms/1

== system controller_dev_sg/Rx_TPCommsControllerSide/CheckCommsTrajectory ==
  WatchdogEmergency : Inport
  WatchdogPerformance : Inport  Port=2
  CheckComms : misc/CheckComms  timeout_s=tPX2CommsTimeout  tS=tS
  CheckComms1 : misc/CheckComms  timeout_s=tPX2CommsTimeout  tS=tS
  Constant10 : Constant  Value=TUMHealthStatus.ERROR  OutDataTypeStr=Enum: TUMHealthStatus  SampleTime=-1
  Constant3 : Constant  Value=TUMHealthStatus.OK  OutDataTypeStr=Enum: TUMHealthStatus  SampleTime=-1
  Logical Operator : Logic  AllPortsSameDT=off  OutDataTypeStr=boolean
  Switch : Switch  Criteria=u2 > Threshold
  HealthStatus : Outport
  wires:
  Constant10/1 -> Switch/3
  Logical Operator/1 -> Switch/2
  CheckComms/1 -> Logical Operator/1
  CheckComms1/1 -> Logical Operator/2
  Constant3/1 -> Switch/1
  Switch/1 -> HealthStatus/1
  WatchdogEmergency/1 -> CheckComms1/1
  WatchdogPerformance/1 -> CheckComms/1

== system controller_dev_sg/Rx_TPCommsControllerSide/Clock ==
  Counter Free-Running : simulink/Sources/Counter Free-Running  NumBits=32  tsamp=tS
  Data Type Conversion : DataTypeConversion  OutDataTypeStr=double  SaturateOnIntegerOverflow=on
  Gain : Gain  Gain=tS
  Time_s : Outport
  wires:
  Counter Free-Running/1 -> Data Type Conversion/1
  Gain/1 -> Time_s/1
  Data Type Conversion/1 -> Gain/1

== system controller_dev_sg/Rx_TPCommsControllerSide/ReadBehaviorStateMachinePackage ==
  Raw Data : Inport
  Enable : EnablePort
  Byte Unpack : etargetslib/Byte Unpack  dimensions={[1], [1], [1]}  datatypes={'uint16', 'uint16', 'uint32'}  byteAlign=1
  Data Type Conversion : DataTypeConversion  OutDataTypeStr=Enum: TUMStrategyState  SaturateOnIntegerOverflow=on
  UTC : Outport
  Strategy_Status : Outport  Port=2  OutDataTypeStr=Enum: TUMStrategyState
  Watchdog : Outport  Port=3
  wires:
  Byte Unpack/1 -> Data Type Conversion/1
  Data Type Conversion/1 -> Strategy_Status/1
  Byte Unpack/2 -> Watchdog/1
  Raw Data/1 -> Byte Unpack/1
  Byte Unpack/3 -> UTC/1

== system controller_dev_sg/Rx_TPCommsControllerSide/ReadBehaviorStatemachine1 ==
  Input : Inport
  Compare To Constant : simulink/Logic and Bit Operations/Compare To Constant  Priority=1  relop===  const=8  OutDataTypeStr=boolean
  Min. do-while count : Constant  OutDataTypeStr=int8  SampleTime=-1
  Subtrat : Sum  Inputs=+-
  Terminator : Terminator
  UDP Receive : xpcrtudplib/UDP Receive  ipAddressVal=10.0.1.0  localPort=BehaviorStatemachineRcv_Port  rcvWidth=8  rcvFmAny=off  fmAddress=10.0.2.0  rcvMulticast=off  multicastAddress={}  maxUDPQueue=8  sampleTime=-1
      settings: SourceProductName=Simulink Real-Time
  While Iterator : WhileIterator  WhileBlockType=do-while  ShowIterationPort=on  OutputDataType=int16
  Data : Outport
  NumMsg : Outport  Port=2
  wires:
  Compare To Constant/1 -> While Iterator/1
  UDP Receive/2 -> Compare To Constant/1
  While Iterator/1 -> Subtrat/1
  Min. do-while count/1 -> Subtrat/2
  UDP Receive/1 -> Data/1
  Subtrat/1 -> NumMsg/1  "num msgs this timestep"
  Input/1 -> Terminator/1

== system controller_dev_sg/Rx_TPCommsControllerSide/ReadEmergencyTrajectory1 ==
  Input : Inport
  Compare To Constant : simulink/Logic and Bit Operations/Compare To Constant  relop===  const=4*7*50+2*4  OutDataTypeStr=boolean
  Min. do-while count : Constant  OutDataTypeStr=int8  SampleTime=-1
  Subtrat : Sum  Inputs=+-
  Terminator : Terminator
  UDP Receive : xpcrtudplib/UDP Receive  ipAddressVal=10.0.1.0  localPort=EmergencyPathRcv_Port  rcvWidth=4*7*50+2*4  rcvFmAny=off  fmAddress=10.0.2.0  rcvMulticast=off  multicastAddress={}  maxUDPQueue=8  sampleTime=-1
      settings: SourceProductName=Simulink Real-Time
  While Iterator : WhileIterator  WhileBlockType=do-while  ShowIterationPort=on  OutputDataType=int16
  Data : Outport
  NumMsg : Outport  Port=2
  wires:
  UDP Receive/2 -> Compare To Constant/1
  While Iterator/1 -> Subtrat/1
  Min. do-while count/1 -> Subtrat/2
  UDP Receive/1 -> Data/1
  Compare To Constant/1 -> While Iterator/1
  Subtrat/1 -> NumMsg/1  "num msgs this timestep"
  Input/1 -> Terminator/1

== system controller_dev_sg/Rx_TPCommsControllerSide/ReadEmergencyTrajectoryPackage ==
  Raw Data : Inport
  Enable : EnablePort
  Bus Creator2 : BusCreator  Inputs=10  OutDataTypeStr=Bus: Trajectory
      settings: InheritFromInputs=off
  Byte Unpack : etargetslib/Byte Unpack  dimensions={[1], [1], [50], [50], [50], [50], [50], [50],[50]}  datatypes={'uint32', 'uint32', 'single', 'single', 'single', 'single', 'single', 'single', 'single'}  byteAlign=1
  Constant2 : Constant  Value=zeros(50, 1)
  Data Type Conversion{,1..6} (7 alike) : DataTypeConversion
  TargetTrajectory : Outport  OutDataTypeStr=Bus: Trajectory
  wires:
  Byte Unpack/1 -> Bus Creator2/1  "LapCnt"
  Byte Unpack/2 -> Bus Creator2/2  "TrajCnt"
  Bus Creator2/1 -> TargetTrajectory/1
  Raw Data/1 -> Byte Unpack/1
  Byte Unpack/3 -> Data Type Conversion/1
  Byte Unpack/4 -> Data Type Conversion1/1
  Constant2/1 -> Bus Creator2/4  "s_glob_m"
  Data Type Conversion/1 -> Bus Creator2/3  "s_loc_m"
  Data Type Conversion1/1 -> Bus Creator2/5  "x_m"
  Data Type Conversion2/1 -> Bus Creator2/6  "y_m"
  Byte Unpack/5 -> Data Type Conversion2/1
  Data Type Conversion3/1 -> Bus Creator2/7  "psi_rad"
  Data Type Conversion4/1 -> Bus Creator2/8  "kappa_radpm"
  Data Type Conversion5/1 -> Bus Creator2/9  "v_mps"
  Data Type Conversion6/1 -> Bus Creator2/10  "ax_mps2"
  Byte Unpack/6 -> Data Type Conversion3/1
  Byte Unpack/7 -> Data Type Conversion4/1
  Byte Unpack/8 -> Data Type Conversion5/1
  Byte Unpack/9 -> Data Type Conversion6/1

== system controller_dev_sg/Rx_TPCommsControllerSide/ReadPerformanceTrajectory1 ==
  Input : Inport
  Compare To Constant : simulink/Logic and Bit Operations/Compare To Constant  relop===  const=4*7*50+3*4+2  OutDataTypeStr=boolean
  Min. do-while count : Constant  OutDataTypeStr=int8  SampleTime=-1
  Subtrat : Sum  Inputs=+-
  Terminator : Terminator
  UDP Receive : xpcrtudplib/UDP Receive  ipAddressVal=10.0.1.0  localPort=PerformanceTrajectoryRcv_Port  rcvWidth=4*7*50+2*4  rcvFmAny=off  fmAddress=10.0.2.0  rcvMulticast=off  multicastAddress={}  maxUDPQueue=8  sampleTime=-1
      settings: SourceProductName=Simulink Real-Time
  While Iterator : WhileIterator  WhileBlockType=do-while  ShowIterationPort=on  OutputDataType=int16
  Data : Outport
  NumMsg : Outport  Port=2
  wires:
  Compare To Constant/1 -> While Iterator/1
  UDP Receive/2 -> Compare To Constant/1
  UDP Receive/1 -> Data/1
  While Iterator/1 -> Subtrat/1
  Min. do-while count/1 -> Subtrat/2
  Subtrat/1 -> NumMsg/1  "num msgs this timestep"
  Input/1 -> Terminator/1

== system controller_dev_sg/Rx_TPCommsControllerSide/ReadPerformanceTrajectoryPackage ==
  Raw Data : Inport
  Enable : EnablePort
  Bus Creator2 : BusCreator  Inputs=10  OutDataTypeStr=Bus: Trajectory
      settings: InheritFromInputs=off
  Byte Unpack : etargetslib/Byte Unpack  dimensions={[1], [1], [50], [50], [50], [50], [50], [50],[50]}  datatypes={'uint32', 'uint32', 'single', 'single', 'single', 'single', 'single', 'single', 'single'}  byteAlign=1
  Constant2 : Constant  Value=zeros(50, 1)
  Data Type Conversion{,1..6} (7 alike) : DataTypeConversion
  TargetTrajectory : Outport  OutDataTypeStr=Bus: Trajectory
  wires:
  Byte Unpack/1 -> Bus Creator2/1  "LapCnt"
  Byte Unpack/2 -> Bus Creator2/2  "TrajCnt"
  Bus Creator2/1 -> TargetTrajectory/1
  Raw Data/1 -> Byte Unpack/1
  Byte Unpack/3 -> Data Type Conversion/1
  Byte Unpack/4 -> Data Type Conversion1/1
  Constant2/1 -> Bus Creator2/4  "s_glob_m"
  Data Type Conversion/1 -> Bus Creator2/3  "s_loc_m"
  Data Type Conversion1/1 -> Bus Creator2/5  "x_m"
  Data Type Conversion2/1 -> Bus Creator2/6  "y_m"
  Byte Unpack/5 -> Data Type Conversion2/1
  Data Type Conversion3/1 -> Bus Creator2/7  "psi_rad"
  Data Type Conversion4/1 -> Bus Creator2/8  "kappa_radpm"
  Data Type Conversion5/1 -> Bus Creator2/9  "v_mps"
  Data Type Conversion6/1 -> Bus Creator2/10  "ax_mps2"
  Byte Unpack/6 -> Data Type Conversion3/1
  Byte Unpack/7 -> Data Type Conversion4/1
  Byte Unpack/8 -> Data Type Conversion5/1
  Byte Unpack/9 -> Data Type Conversion6/1

== system controller_dev_sg/Rx_TPCommsTPSide/ReadBehaviorStateMachine ==
  Compare To Constant : simulink/Logic and Bit Operations/Compare To Constant  relop===  const=8  OutDataTypeStr=boolean
  Min. do-while count : Constant  OutDataTypeStr=int8  SampleTime=-1
  Subtrat : Sum  Inputs=+-
  UDP Receive : xpcrtudplib/UDP Receive  ipAddressVal=10.0.2.0  localPort=BehaviorStatemachineSend_Port  rcvWidth=8  rcvFmAny=off  fmAddress=10.0.1.0  rcvMulticast=off  multicastAddress={}  maxUDPQueue=8  sampleTime=-1
      settings: SourceProductName=Simulink Real-Time
  While Iterator : WhileIterator  WhileBlockType=do-while  ShowIterationPort=on  OutputDataType=int16
  Data : Outport
  NumMsg : Outport  Port=2
  wires:
  Compare To Constant/1 -> While Iterator/1
  UDP Receive/2 -> Compare To Constant/1
  While Iterator/1 -> Subtrat/1
  Min. do-while count/1 -> Subtrat/2
  Subtrat/1 -> NumMsg/1  "num msgs this timestep"
  UDP Receive/1 -> Data/1

== system controller_dev_sg/Rx_TPCommsTPSide/ReadBehaviorStateMachinePackage ==
  Raw Data : Inport
  Enable : EnablePort
  Byte Unpack : etargetslib/Byte Unpack  dimensions={[1], [1], [1]}  datatypes={'uint16', 'uint32', 'uint16'}  byteAlign=1
  Data Type Conversion : DataTypeConversion  OutDataTypeStr=Enum: TUMVehicleState  SaturateOnIntegerOverflow=on
  Terminator : Terminator
  TUMVehicleState : Outport
  ErrorCode : Outport  Port=2
  wires:
  Byte Unpack/1 -> Data Type Conversion/1
  Data Type Conversion/1 -> TUMVehicleState/1
  Byte Unpack/2 -> ErrorCode/1
  Raw Data/1 -> Byte Unpack/1
  Byte Unpack/3 -> Terminator/1

== system controller_dev_sg/Rx_TPCommsTPSide/ReadTrajectoryGeneration ==
  Compare To Constant : simulink/Logic and Bit Operations/Compare To Constant  relop===  const=25  OutDataTypeStr=boolean
  Min. do-while count : Constant  OutDataTypeStr=int8  SampleTime=-1
  Subtrat : Sum  Inputs=+-
  UDP Receive : xpcrtudplib/UDP Receive  ipAddressVal=10.0.2.0  localPort=TrajectoryGenerationSend_Port  rcvWidth=25  rcvFmAny=off  fmAddress=10.0.1.0  rcvMulticast=off  multicastAddress={}  maxUDPQueue=8  sampleTime=-1
      settings: SourceProductName=Simulink Real-Time
  While Iterator : WhileIterator  WhileBlockType=do-while  ShowIterationPort=on  OutputDataType=int16
  Data : Outport
  NumMsg : Outport  Port=2
  wires:
  Compare To Constant/1 -> While Iterator/1
  UDP Receive/2 -> Compare To Constant/1
  While Iterator/1 -> Subtrat/1
  Min. do-while count/1 -> Subtrat/2
  Subtrat/1 -> NumMsg/1  "num msgs this timestep"
  UDP Receive/1 -> Data/1

== system controller_dev_sg/Rx_TPCommsTPSide/ReadTrajectoryGeneration1 ==
  Raw Data : Inport
  Enable : EnablePort
  Byte Unpack : etargetslib/Byte Unpack  dimensions={[6], [1]}  datatypes={['single'], 'uint8'}  byteAlign=1
  Data Type Conversion : DataTypeConversion  OutDataTypeStr=double  SaturateOnIntegerOverflow=on
  BDriveMode : Outport
  RcvData : Outport  Port=2  SourceOfInitialOutputValue=Input signal
  wires:
  Byte Unpack/2 -> BDriveMode/1
  Raw Data/1 -> Byte Unpack/1
  Byte Unpack/1 -> Data Type Conversion/1
  Data Type Conversion/1 -> RcvData/1

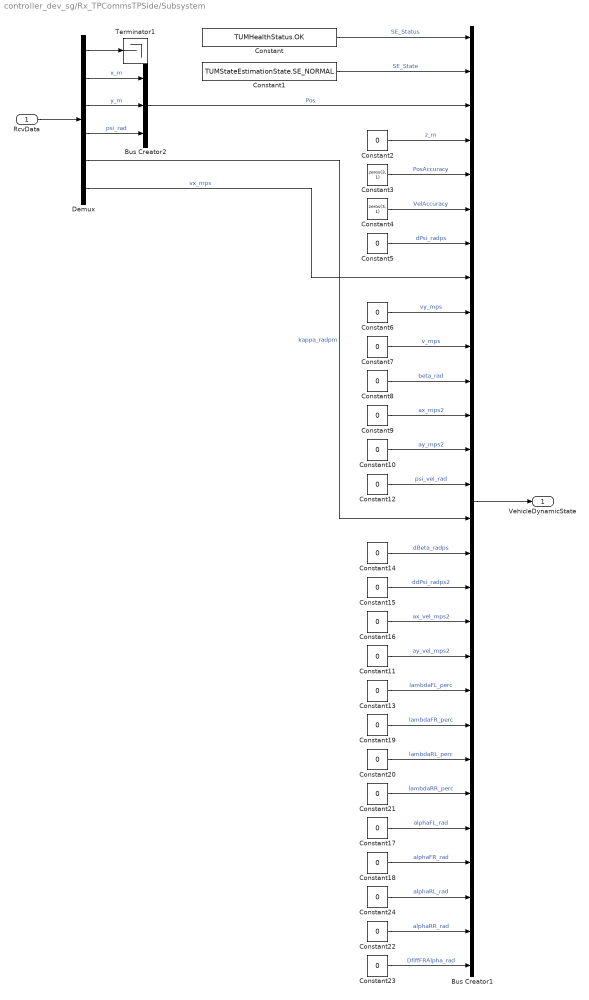
== system controller_dev_sg/Rx_TPCommsTPSide/Subsystem ==
  RcvData : Inport
  Bus Creator1 : BusCreator  Inputs=28
  Bus Creator2 : BusCreator  Inputs=3  OutDataTypeStr=Bus: CartPos
  Constant : Constant  Value=TUMHealthStatus.OK
  Constant1 : Constant  Value=TUMStateEstimationState.SE_NORMAL
  Constant{2,5..24} (21 alike) : Constant  Value=0
  Constant3 : Constant  Value=zeros(3, 1)
  Constant4 : Constant  Value=zeros(3, 1)
  Demux : Demux  Outputs=6
  Terminator1 : Terminator
  VehicleDynamicState : Outport
  wires:
  Constant/1 -> Bus Creator1/1  "SE_Status"
  Constant1/1 -> Bus Creator1/2  "SE_State"
  Constant24/1 -> Bus Creator1/26  "alphaRL_rad"
  Bus Creator1/1 -> VehicleDynamicState/1
  Constant18/1 -> Bus Creator1/25  "alphaFR_rad"
  Demux/6 -> Bus Creator1/8  "vx_mps"
  Demux/2 -> Bus Creator2/1  "x_m"
  Constant12/1 -> Bus Creator1/14  "psi_vel_rad"
  Constant4/1 -> Bus Creator1/6  "VelAccuracy"
  Bus Creator2/1 -> Bus Creator1/3  "Pos"
  Demux/3 -> Bus Creator2/2  "y_m"
  Constant2/1 -> Bus Creator1/4  "z_m"
  Constant7/1 -> Bus Creator1/10  "v_mps"
  Demux/5 -> Bus Creator1/15  "kappa_radpm"
  Constant17/1 -> Bus Creator1/24  "alphaFL_rad"
  Constant13/1 -> Bus Creator1/20  "lambdaFL_perc"
  Constant15/1 -> Bus Creator1/17  "ddPsi_radps2"
  Constant19/1 -> Bus Creator1/21  "lambdaFR_perc"
  Constant14/1 -> Bus Creator1/16  "dBeta_radps"
  Constant16/1 -> Bus Creator1/18  "ax_vel_mps2"
  Constant6/1 -> Bus Creator1/9  "vy_mps"
  Constant23/1 -> Bus Creator1/28  "DfiffFRAlpha_rad"
  Demux/4 -> Bus Creator2/3  "psi_rad"
  Constant21/1 -> Bus Creator1/23  "lambdaRR_perc"
  Demux/1 -> Terminator1/1
  Constant8/1 -> Bus Creator1/11  "beta_rad"
  Constant3/1 -> Bus Creator1/5  "PosAccuracy"
  Constant5/1 -> Bus Creator1/7  "dPsi_radps"
  Constant22/1 -> Bus Creator1/27  "alphaRR_rad"
  Constant10/1 -> Bus Creator1/13  "ay_mps2"
  RcvData/1 -> Demux/1
  Constant20/1 -> Bus Creator1/22  "lambdaRL_perc"
  Constant9/1 -> Bus Creator1/12  "ax_mps2"
  Constant11/1 -> Bus Creator1/19  "ay_vel_mps2"
